simulink library "fp_utilities"  (R2022b)
settings: Solver=VariableStepAuto  StartTime=0.0  StopTime=10.0  RelTol=1e-3
libraries: spsCurrentMeasurementLib x1, spsVoltageMeasurementLib x1
settings Model: Creator=Javnson  LastModifiedBy=Javnson

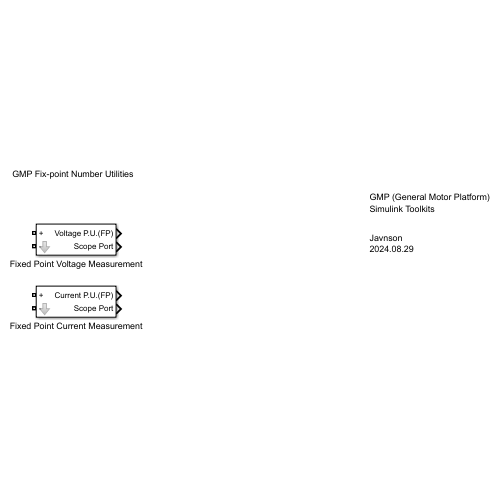
[thumbnail: Simulink's stored preview of the top-level diagram]
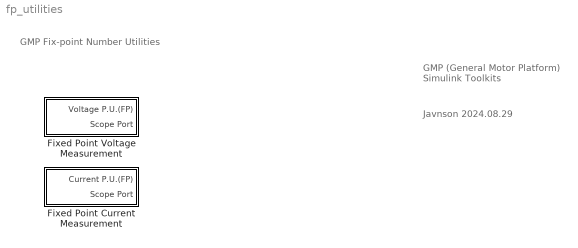
== system fp_utilities ==
  note: GMP Fix-point Number Utilities
  note: GMP (General Motor Platform)
      | Simulink Toolkits
  note: Javnson
      | 2024.08.29
  Fixed Point Current Measurement : Subsystem  mask{PerUnit_Base=60, Q_VALUE=24}
      mask prompts: PerUnit_Base "PerUnit_Base (A) :"; Q_VALUE "Q_num"
      mask DialogControl DescGroupVar Prompt: Fixed Point Voltage Measurement
      mask DialogControl DescTextVar Prompt: Measure a voltage value and transfer the real value (double type) to perunit value(int32_t).
      mask DialogControl Control2 Prompt: Parameter per unit base value:
      mask DialogControl Control3 Prompt: Fixed-point Number Q value:
  Fixed Point Voltage Measurement : Subsystem  mask{PerUnit_Base=60, Q_VALUE=24}
      mask prompts: PerUnit_Base "PerUnit_Base (V) :"; Q_VALUE "Q_num"
      mask DialogControl DescGroupVar Prompt: Fixed Point Voltage Measurement
      mask DialogControl DescTextVar Prompt: Measure a voltage value and transfer the real value (double type) to perunit value(int32_t).
      mask DialogControl Control2 Prompt: Parameter per unit base value:
      mask DialogControl Control3 Prompt: Fixed-point Number Q value:

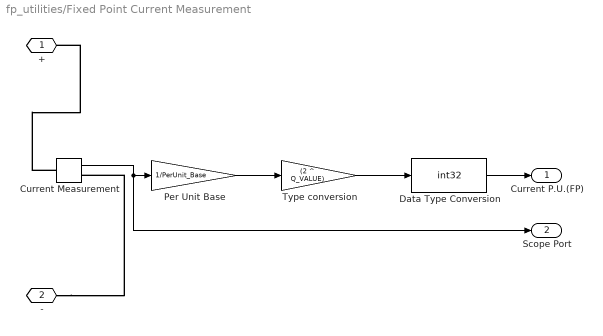
== system fp_utilities/Fixed Point Current Measurement ==
  Current Measurement : spsCurrentMeasurementLib/Current Measurement  PhasorSimulation=off  OutputType=Complex  PSBequivalent=0
  Data Type Conversion : DataTypeConversion  OutDataTypeStr=int32  ConvertRealWorld=Stored Integer (SI)  SaturateOnIntegerOverflow=off  RndMeth=Floor  LockScale=on
  Per Unit Base : Gain  Gain=1/PerUnit_Base
  Type conversion : Gain  Gain=(2 ^ Q_VALUE)
  + : PMIOPort  Side=Left
  - : PMIOPort  Port=2  Side=Left
  Current P.U.(FP) : Outport
  Scope Port : Outport  Port=2
  wires:
  Per Unit Base/1 -> Type conversion/1
  Type conversion/1 -> Data Type Conversion/1
  Data Type Conversion/1 -> Current P.U.(FP)/1
  Current Measurement/1 -> Scope Port/1, Per Unit Base/1
  connections:
  -/RConn1 -- Current Measurement/RConn1
  Current Measurement/LConn1 -- +/RConn1

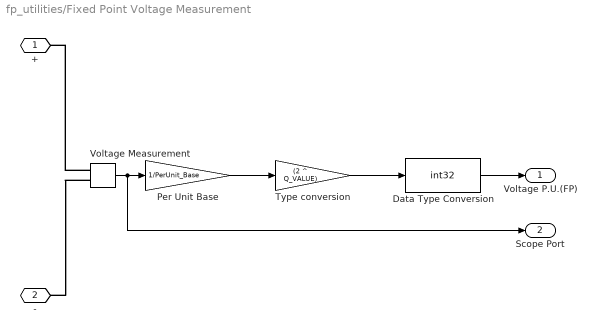
== system fp_utilities/Fixed Point Voltage Measurement ==
  Data Type Conversion : DataTypeConversion  OutDataTypeStr=int32  ConvertRealWorld=Stored Integer (SI)  SaturateOnIntegerOverflow=off  RndMeth=Floor  LockScale=on
  Per Unit Base : Gain  Gain=1/PerUnit_Base
  Type conversion : Gain  Gain=(2 ^ Q_VALUE)
  Voltage Measurement : spsVoltageMeasurementLib/Voltage Measurement  PhasorSimulation=off  OutputType=Complex  PSBequivalent=0
  + : PMIOPort  Side=Left
  - : PMIOPort  Port=2  Side=Left
  Voltage P.U.(FP) : Outport
  Scope Port : Outport  Port=2
  wires:
  Per Unit Base/1 -> Type conversion/1
  Type conversion/1 -> Data Type Conversion/1
  Data Type Conversion/1 -> Voltage P.U.(FP)/1
  Voltage Measurement/1 -> Scope Port/1, Per Unit Base/1
  connections:
  Voltage Measurement/LConn2 -- -/RConn1
  Voltage Measurement/LConn1 -- +/RConn1
